simulink model "p1a_model"  (Simulink 8.7)
settings: Solver=FixedStepAuto  StartTime=0.0  StopTime=8  FixedStep=0.5  RelTol=1e-3
settings Model: Creator=eispin  LastModifiedBy=eispin
settings DataIOCC: LimitDataPoints=off  SaveFormat=Dataset
settings DebuggingCC: UnderspecifiedInitializationDetection=Simplified  MergeDetectMultiDrivingBlocksExec=error
settings HardwareCC: ProdBitPerPointer=64  ProdLargestAtomicFloat=Float  ProdIntDivRoundTo=Zero  ProdEndianess=LittleEndian  ProdWordSize=64  ProdHWDeviceType=Intel->x86-64 (Windows64)
settings ModelReferenceCC: PropagateSignalLabelsOutOfModel=on
settings ConfigComp: CovModelRefEnable=off

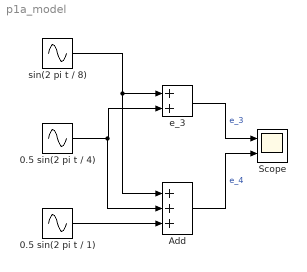
== system p1a_model ==
  0.5 sin(2 pi t / 1) : Sin  Amplitude=0.5  Frequency=2 * pi / 1  SampleTime=0
  0.5 sin(2 pi t / 4) : Sin  Amplitude=0.5  Frequency=2 * pi / 4  SampleTime=0
  Add : Sum  Inputs=+++
  Scope : Scope  NumInputPorts=2
  e_3 : Sum
  sin(2 pi t / 8) : Sin  Frequency=2 * pi / 8  SampleTime=0
  wires:
  sin(2 pi t / 8)/1 -> Add/1, e_3/1
  0.5 sin(2 pi t / 4)/1 -> Add/2, e_3/2
  0.5 sin(2 pi t / 1)/1 -> Add/3
  e_3/1 -> Scope/1  "e_3"
  Add/1 -> Scope/2  "e_4"
